simulink model "Main"  (R2020a)
settings: Solver=FixedStepDiscrete  StartTime=0.0  StopTime=Inf  RelTol=1e-3  EnableMultiTasking=on
undefined symbols (not defined in the file or in its folder): IO397
libraries: slrtlib x4, speedgoatlib_fpga_analog_io x2, speedgoatlib_fpga x1
settings Model: SimulationMode=external  Creator=ejgonzal  LastModifiedBy=ejgonzal
settings SolverCC: ConcurrentTasks=on  AutoInsertRateTranBlk=on
settings DataIOCC: SaveFormat=StructureWithTime  SaveOutput=off  SignalLogging=off  DSMLogging=off  SaveTime=off  ReturnWorkspaceOutputs=off
settings OptimizationCC: BlockReduction=off  OptimizeBlockIOStorage=off
settings HardwareCC: ProdBitPerPointer=32  ProdBitPerSizeT=32  ProdBitPerPtrDiffT=32  ProdLargestAtomicFloat=None  ProdWordSize=32  ProdLongLongMode=on  ProdHWDeviceType=Generic->32-bit x86 compatible
settings RTWCC: Description=Simulink Real-Time  SystemTargetFile=slrt.tlc  TLCOptions=-axPCMaxOverloads=1000 -axPCOverLoadLen=1 -axPCStartupFlag=5  TemplateMakefile=slrt_default_tmf  RTWVerbose=off  CodeExecutionProfiling=on  RTWCompilerOptimization=on
settings SimulinkRealTimeCC: SupportVariableSizeSignals=on  RL32LogTETModifier=off  xPCConcurrentTasks=on

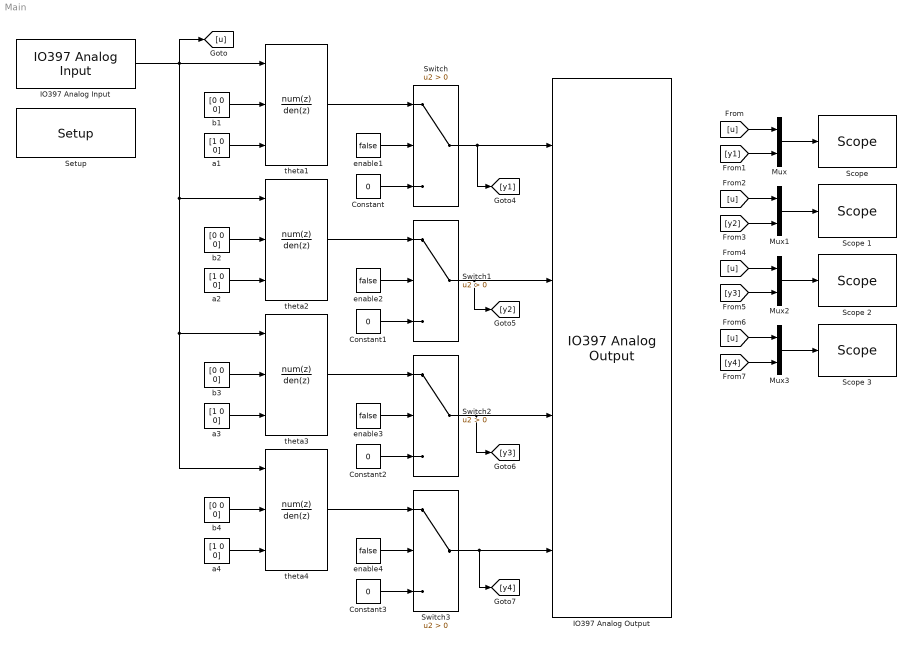
== system Main ==
  Constant{,1..3} (4 alike) : Constant  Value=0  SampleTime=-1
  IO397 Analog Input : speedgoatlib_fpga_analog_io/IO397 Analog Input  id=1  chan=1  range=+-10 V  trigger=Initiator  ts=1/16e3  pciSlot=-1  board=IO397-50k
      settings: SourceProductName=Simulink Real-Time: Speedgoat I/O Blockset
  IO397 Analog Output : speedgoatlib_fpga_analog_io/IO397 Analog Output  id=1  chan=1:4  initVal=0  resetVal=0  ts=-1  pciSlot=-1  board=IO397-50k  span=+-10 V
      settings: SourceProductName=Simulink Real-Time: Speedgoat I/O Blockset
  Mux{,1..3} (4 alike) : Mux  Inputs=2
  "Scope " : slrtlib/Displays and Logging/Scope   scopeno=1  scopetype=Target  autostart=on  viewmode=Graphical redraw  formatstr='%15.6f'  grid=on  ylimits=[-2, 2]  nosamples=250  noprepostsamples=0  interleave=1  triggermode=FreeRun  triggersignal=1  trigsignalfromport=off  triggerlevel=0.0  triggerslope=Either  triggerscope=1  triggersample=0  filename=data.dat  mode=Lazy  writesize=512  autorestart=off  dynamicfilemode=off  maxwritefilesize=512*1024^2
  Scope 1 : slrtlib/Displays and Logging/Scope   scopeno=2  scopetype=Target  autostart=on  viewmode=Graphical redraw  formatstr='%15.6f'  grid=on  ylimits=[-2, 2]  nosamples=250  noprepostsamples=0  interleave=1  triggermode=FreeRun  triggersignal=1  trigsignalfromport=off  triggerlevel=0.0  triggerslope=Either  triggerscope=1  triggersample=0  filename=data.dat  mode=Lazy  writesize=512  autorestart=off  dynamicfilemode=off  maxwritefilesize=512*1024^2
  Scope 2 : slrtlib/Displays and Logging/Scope   scopeno=3  scopetype=Target  autostart=on  viewmode=Graphical redraw  formatstr='%15.6f'  grid=on  ylimits=[-2, 2]  nosamples=250  noprepostsamples=0  interleave=1  triggermode=FreeRun  triggersignal=1  trigsignalfromport=off  triggerlevel=0.0  triggerslope=Either  triggerscope=1  triggersample=0  filename=data.dat  mode=Lazy  writesize=512  autorestart=off  dynamicfilemode=off  maxwritefilesize=512*1024^2
  Scope 3 : slrtlib/Displays and Logging/Scope   scopeno=4  scopetype=Target  autostart=on  viewmode=Graphical redraw  formatstr='%15.6f'  grid=on  ylimits=[-2, 2]  nosamples=250  noprepostsamples=0  interleave=1  triggermode=FreeRun  triggersignal=1  trigsignalfromport=off  triggerlevel=0.0  triggerslope=Either  triggerscope=1  triggersample=0  filename=data.dat  mode=Lazy  writesize=512  autorestart=off  dynamicfilemode=off  maxwritefilesize=512*1024^2
  Setup : speedgoatlib_fpga/Setup/Setup  board=IO397-50k  id=1  device_id=1  frontIO=None  rearIO=None  bitstreamFile=speedgoat_IO397_50k_all_io.mat  rev=1.0  timestamp_string=21/11/18 14:52:53  fpgaFreq=75 MHz  fpgaTick=13.33 ns  ProgSpiFlash=off  ProgBPIFlash=off  pciSlot=-1  PullRPort0=pull-up 3.3V  VioPort0=3.3V  PullRPort1=pull-up 3.3V  VioPort1=3.3V  PullRPort2=pull-up 3.3V  VioPort2=3.3V  PullRPort3=pull-up 3.3V  VioPort3=3.3V  PullRPort4=pull-up 3.3V  VioPort4=3.3V  PullRPort5=pull-up 3.3V  VioPort5=3.3V  PullRPort6=pull-up 3.3V  VioPort6=3.3V  PullRPort15=pull-up 3.3V  PullRPort31=pull-up 3.3V  PullRPort47=pull-up 3.3V  PullRPort63=pull-up 3.3V
      settings: SourceProductName=Simulink Real-Time: Speedgoat I/O Blockset
  Switch{,1..3} (4 alike) : Switch  Criteria=u2 > Threshold
  a{1..4} (4 alike) : Constant  Value=[1 0 0]  SampleTime=-1
  b{1..4} (4 alike) : Constant  Value=[0 0 0]  SampleTime=-1
  enable{1..4} (4 alike) : Constant  Value=false  SampleTime=-1
  theta{1..4} (4 alike) : DiscreteFilter  NumeratorSource=Input port  Numerator=[0 0 0]  DenominatorSource=Input port  Denominator=[1, 0 0]  a0EqualsOne=on
      settings: InputPortMap=u0,p1,p3
  wires:
  Constant/1 -> Switch/3
  enable1/1 -> Switch/2
  b1/1 -> theta1/2
  a1/1 -> theta1/3
  b2/1 -> theta2/2
  a2/1 -> theta2/3
  a3/1 -> theta3/3
  b3/1 -> theta3/2
  b4/1 -> theta4/2
  a4/1 -> theta4/3
  theta1/1 -> Switch/1
  enable2/1 -> Switch1/2
  Constant1/1 -> Switch1/3
  theta2/1 -> Switch1/1
  enable3/1 -> Switch2/2
  Constant2/1 -> Switch2/3
  theta3/1 -> Switch2/1
  enable4/1 -> Switch3/2
  Constant3/1 -> Switch3/3
  theta4/1 -> Switch3/1
  Switch/1 -> IO397 Analog Output/1, [y1]
  Switch1/1 -> [y2], IO397 Analog Output/2
  Switch2/1 -> [y3], IO397 Analog Output/3
  Switch3/1 -> [y4], IO397 Analog Output/4
  IO397 Analog Input/1 -> theta1/1, [u], theta4/1, theta3/1, theta2/1
  Mux/1 -> "Scope "/1
  [y1] -> Mux/2
  [u] -> Mux/1
  Mux1/1 -> Scope 1/1
  [y2] -> Mux1/2
  [u] -> Mux1/1
  [u] -> Mux2/1
  [y3] -> Mux2/2
  Mux2/1 -> Scope 2/1
  Mux3/1 -> Scope 3/1
  [y4] -> Mux3/2
  [u] -> Mux3/1
